simulink model "pendulumc_2"  (R2020a)
settings: Solver=VariableStepAuto  StartTime=0.0  StopTime=50  RelTol=1e-3
values from neighbouring files (symbols this model uses):
  b = 0    [scriptpendulumc.m]
  g = 9.82    [scriptpendulumc.m]
  l = 1    [scriptpendulumc.m]
  m = 1    [scriptpendulumc.m]
undefined symbols (not defined in the file or in its folder): theta0
libraries: simulink x2
settings Model: Creator=mumun  LastModifiedBy=mumun

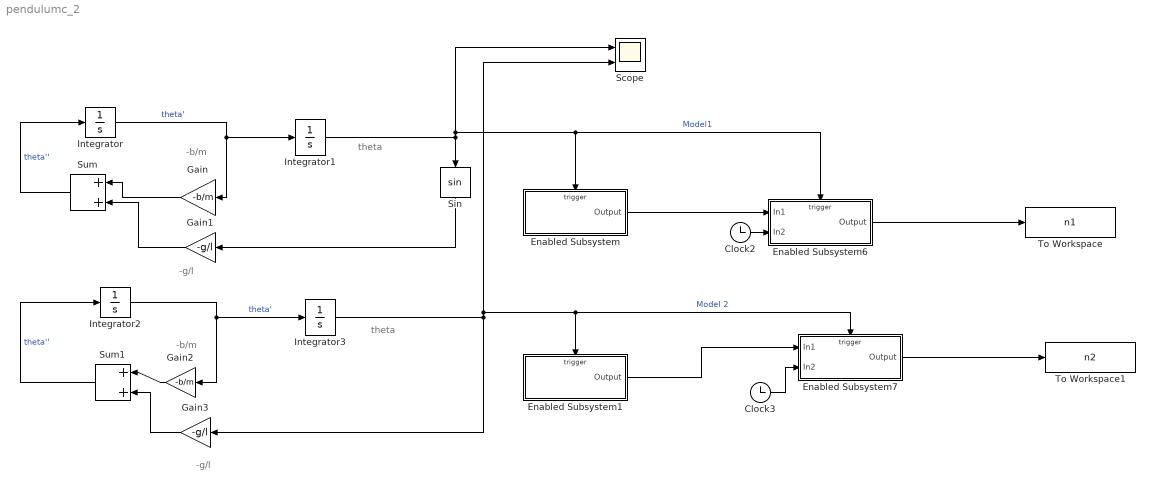
== system pendulumc_2 ==
  note: -g/l
  note: theta
  note: -g/l
  note: -b/m
  note: -b/m
  note: theta
  Clock2 : Clock
  Clock3 : Clock
  Enabled Subsystem : Subsystem  TreatAsAtomicUnit=on
  Enabled Subsystem1 : Subsystem  TreatAsAtomicUnit=on
  Enabled Subsystem6 : Subsystem  TreatAsAtomicUnit=on
  Enabled Subsystem7 : Subsystem  TreatAsAtomicUnit=on
  Gain : Gain  Gain=-b/m
  Gain1 : Gain  Gain=-g/l
  Gain2 : Gain  Gain=-b/m
  Gain3 : Gain  Gain=-g/l
  Integrator : Integrator
  Integrator1 : Integrator  InitialCondition=theta0
  Integrator2 : Integrator
  Integrator3 : Integrator  InitialCondition=theta0
  Scope : Scope  NumInputPorts=2
  Sin : Trigonometry
  Sum : Sum  Inputs=|++
  Sum1 : Sum  Inputs=|++
  To Workspace : ToWorkspace  VariableName=n1  SampleTime=-1
      settings: Save2DSignal=2-D array (concatenate along first dimension)
  To Workspace1 : ToWorkspace  VariableName=n2  SampleTime=-1
      settings: Save2DSignal=2-D array (concatenate along first dimension)
  wires:
  Integrator/1 -> Gain/1, Integrator1/1  "theta'"
  Sin/1 -> Gain1/1
  Gain/1 -> Sum/1
  Gain1/1 -> Sum/2
  Sum/1 -> Integrator/1  "theta''"
  Sum1/1 -> Integrator2/1  "theta''"
  Gain2/1 -> Sum1/1
  Gain3/1 -> Sum1/2
  Integrator2/1 -> Gain2/1, Integrator3/1  "theta'"
  Integrator3/1 -> Enabled Subsystem7/Trigger, Enabled Subsystem1/Trigger, Scope/2, Gain3/1  "Model 2"
  Integrator1/1 -> Scope/1, Enabled Subsystem6/Trigger, Enabled Subsystem/Trigger, Sin/1  "Model1"
  Clock2/1 -> Enabled Subsystem6/2(In2)
  Enabled Subsystem6/1(Output) -> To Workspace/1
  Enabled Subsystem/1(Output) -> Enabled Subsystem6/1(In1)
  Enabled Subsystem7/1(Output) -> To Workspace1/1
  Clock3/1 -> Enabled Subsystem7/2(In2)
  Enabled Subsystem1/1(Output) -> Enabled Subsystem7/1(In1)

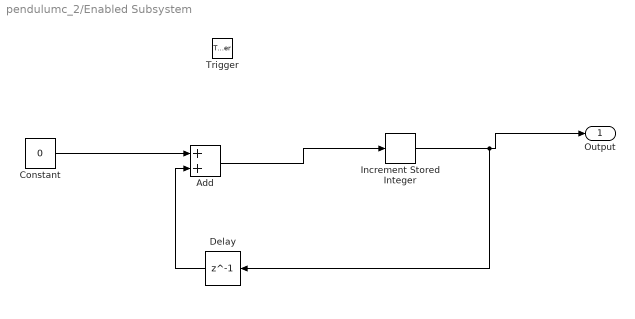
== system pendulumc_2/Enabled Subsystem ==
  Trigger : TriggerPort  VariantControl=Variant  PortDimensions=1
  Add : Sum
  Constant : Constant  Value=0
  Delay : Delay  DelayLength=1
  Increment Stored Integer : simulink/Additional Math & Discrete/Additional Math: Increment - Decrement/Increment Stored Integer
  Output : Outport
  wires:
  Constant/1 -> Add/1
  Add/1 -> Increment Stored Integer/1
  Increment Stored Integer/1 -> Delay/1, Output/1
  Delay/1 -> Add/2

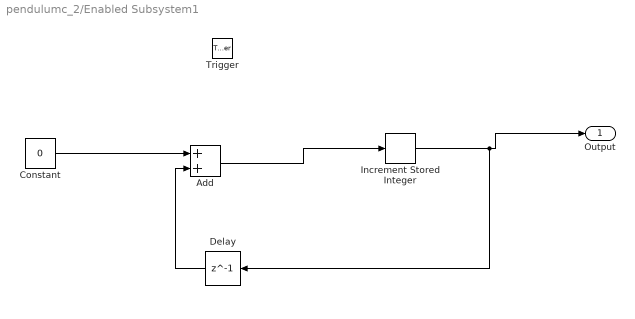
== system pendulumc_2/Enabled Subsystem1 ==
  Trigger : TriggerPort  VariantControl=Variant  PortDimensions=1
  Add : Sum
  Constant : Constant  Value=0
  Delay : Delay  DelayLength=1
  Increment Stored Integer : simulink/Additional Math & Discrete/Additional Math: Increment - Decrement/Increment Stored Integer
  Output : Outport
  wires:
  Constant/1 -> Add/1
  Add/1 -> Increment Stored Integer/1
  Increment Stored Integer/1 -> Delay/1, Output/1
  Delay/1 -> Add/2

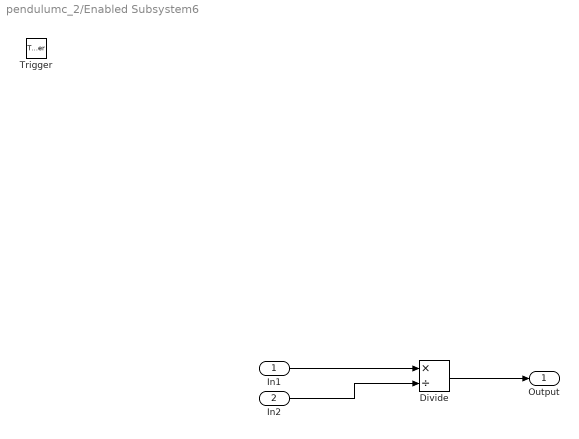
== system pendulumc_2/Enabled Subsystem6 ==
  In1 : Inport
  In2 : Inport  Port=2
  Trigger : TriggerPort  VariantControl=Variant  PortDimensions=1
  Divide : Product  Inputs=*/
  Output : Outport
  wires:
  In1/1 -> Divide/1
  Divide/1 -> Output/1
  In2/1 -> Divide/2

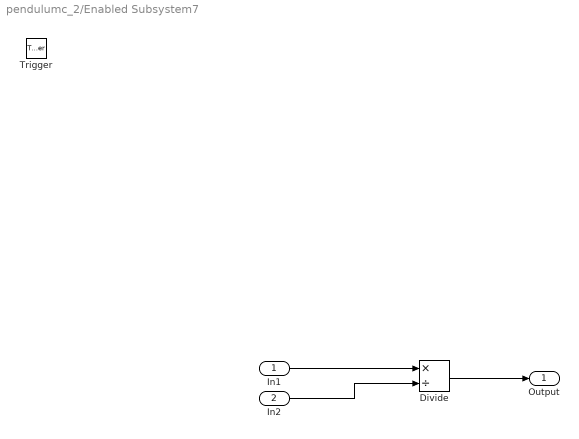
== system pendulumc_2/Enabled Subsystem7 ==
  In1 : Inport
  In2 : Inport  Port=2
  Trigger : TriggerPort  VariantControl=Variant  PortDimensions=1
  Divide : Product  Inputs=*/
  Output : Outport
  wires:
  In1/1 -> Divide/1
  Divide/1 -> Output/1
  In2/1 -> Divide/2
